simulink model "PV_MODEL4"  (R2023a)
settings: Solver=ode23tb  StartTime=0.0  StopTime=1  RelTol=1e-3
PreLoadFcn:
  | Nss=2;
  | Npp=2;
  | Ki=0.015;
  | Kv=-.1;
  | Tn=25;
  | Vocn=32.9;
  | Iscn=8.21;
  | Rs=.001;
  | Ipvn=8.214;
  | k= (1.38)*(1e-23);
  | Tn=298.15;
  | Gn=1000;
  | a=1.3;
  | q= (1.60) * (1e-19);
  | Ns=54;
  | Rp=600.405;Nss=2;
  | Npp=2;
  | Ki=0.015;
  | Kv=-.1;
  | Tn=25;
  | Vocn=32.9;
  | Iscn=8.21;
  | Rs=.001;
  | Ipvn=8.214;
  | k= (1.38)*(1e-23);
  | Tn=298.15;
  | Gn=1000;
  | a=1.3;
  | q= (1.60) * (1e-19);
  | Ns=54;
  | Rp=600.405;
libraries: spsSeriesRLCBranchLib x4, powerlib_extras x2, spsVoltageMeasurementLib x2, spsCurrentMeasurementLib x1, spsDiodeLib x1, spsIGBTLib x1, simulink x1, spsPVArrayLib x1, sps_lib x1
settings Model: Creator=dell  LastModifiedBy=ankit
settings SolverCC: AlgebraicLoopSolver=TrustRegion
settings DataIOCC: LimitDataPoints=on  SaveFormat=Array  SignalLoggingSaveFormat=ModelDataLogs  ReturnWorkspaceOutputs=off
settings OptimizationCC: BlockReduction=off  BooleanDataType=off  LifeSpan=inf
settings DebuggingCC: SaveWithParameterizedLinksMsg=none  UnderspecifiedInitializationDetection=Classic  MergeDetectMultiDrivingBlocksExec=none  SignalResolutionControl=TryResolveAllWithWarning  MultiTaskDSMMsg=warning  MultiTaskCondExecSysMsg=none  UnconnectedInputMsg=warning  UnconnectedOutputMsg=warning  UnconnectedLineMsg=warning  StateNameClashWarn=warning  SFUnexpectedBacktrackingDiag=warning  SFNoUnconditionalDefaultTransitionDiag=warning  SFExecutionAtInitializationDiag=none  ArithmeticOperatorsInVariantConditions=warning
settings HardwareCC: ProdBitPerPointer=32  ProdBitPerSizeT=32  ProdBitPerPtrDiffT=32  ProdLargestAtomicFloat=None  ProdIntDivRoundTo=Undefined  ProdEndianess=Unspecified  ProdWordSize=32  ProdHWDeviceType=32-bit Generic  TargetUnknown=on
settings ModelReferenceCC: PropagateSignalLabelsOutOfModel=off
settings SFSimCC: SimUseLocalCustomCode=off  CustomCodeUndefinedFunction=UseInterfaceOnly
settings RTWCC: RTWUseLocalCustomCode=off
settings CodeAppCC: StateflowObjectComments=on
settings GRTTargetCC: TargetLangStandard=C89/C90 (ANSI)
settings ConfigComp: CovMetricSettings=dw  CovSaveCumulativeToWorkspaceVar=on  CovSaveSingleToWorkspaceVar=on  CovExternalEMLEnable=off
settings SimscapeCC: SimscapeNormalizeSystem=off

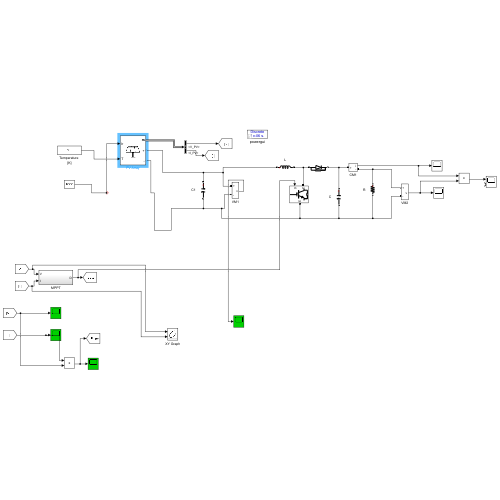
[thumbnail: Simulink's stored preview of the top-level diagram]
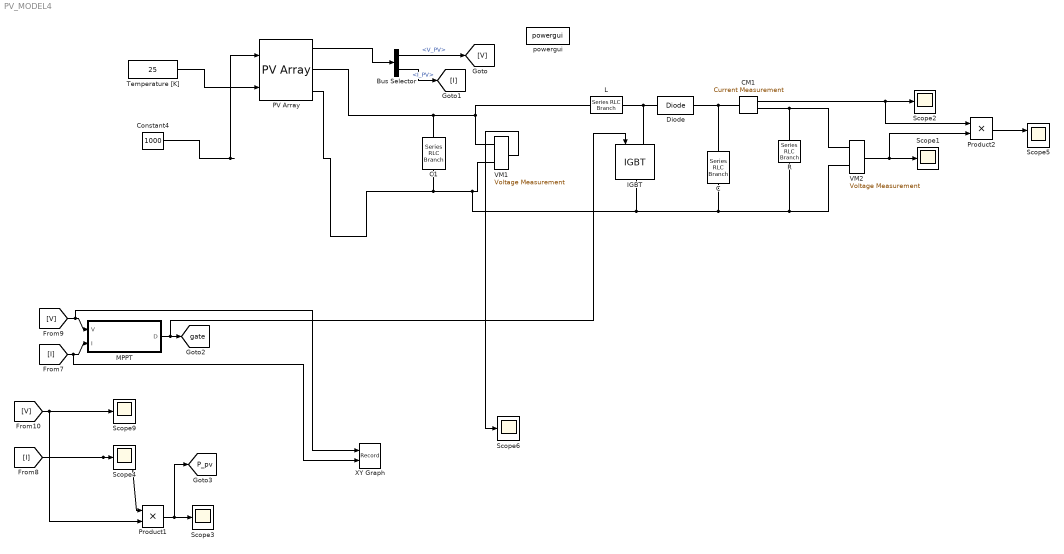
== system PV_MODEL4 ==
  Bus Selector : BusSelector  OutputSignals=V_PV,I_PV
  C : spsSeriesRLCBranchLib/Series RLC Branch  LConnTagsString=__new0  RConnTagsString=__new0  BranchType=C  Resistance=0.01  Inductance=1.0  SetiL0=off  InitialCurrent=0  Capacitance=20e-6  Setx0=off  InitialVoltage=200  Measurements=None
  C1 : spsSeriesRLCBranchLib/Series RLC Branch  LConnTagsString=__new0  RConnTagsString=__new0  BranchType=C  Resistance=0.01  Inductance=1.0  SetiL0=off  InitialCurrent=0  Capacitance=10e-6  Setx0=off  InitialVoltage=200  Measurements=None
  CM1 : spsCurrentMeasurementLib/Current Measurement  Tag=PoWeRsYsTeMmEaSuReMeNt  PhasorSimulation=off  OutputType=Magnitude  PSBequivalent=0
      settings: AttributesFormatString=\n
  Constant4 : Constant  Value=1000
  Diode : spsDiodeLib/Diode  Ron=0.001  Lon=0  Vf=0.8  IC=0  UseSnubber=off  Rs=500  Cs=250e-9  Measurements=off
      settings: AttributesFormatString=\n
  IGBT : spsIGBTLib/IGBT  Ron=0.001  Lon=0  Vf=1  Tf=1e-6  Tt=2e-6  IC=0  Rs=1e5  Cs=inf  Measurements=off
  L : spsSeriesRLCBranchLib/Series RLC Branch  LConnTagsString=__new0  RConnTagsString=__new0  BranchType=L  Resistance=1.0  Inductance=3e-3  SetiL0=off  InitialCurrent=0  Capacitance=1.0  Setx0=off  InitialVoltage=0  Measurements=None
  MPPT : Subsystem
  PV Array : spsPVArrayLib/PV Array  Npar=2  Nser=2  PlotType=array @ 1000 W/m2 & specified temperatures  S_vec="[ 1000  500  100 ]"  Temp_C_vec="[ 25 25  ]"  ModuleName=User-defined  PlotWhenSelected=off  Pm=213.15  Ncell=60  Voc=32.8  Isc=8.21  Vm=29  Im=7.35  beta_Voc_pc=-0.36099  alpha_Isc_pc=0.102  beta_Voc=-0.1184  alpha_Isc=0.0083742  IL=8.2101  I0=1.1241e-09  nI=1.0005  Rsh=67.4422  Rs=0.17921  RobustModel=off  RobustCellTemperature=313.3991  BAL=on  Tc=1e-6  Tfilter=5e-5
  Product1 : Product  RndMeth=Zero
  Product2 : Product  RndMeth=Zero
  R : spsSeriesRLCBranchLib/Series RLC Branch  LConnTagsString=__new0  RConnTagsString=__new0  BranchType=R  Resistance=100  Inductance=1.0  SetiL0=off  InitialCurrent=0  Capacitance=1.0  Setx0=off  InitialVoltage=0  Measurements=None
  Scope{1..4,6,9} (6 alike) : Scope
  Scope5 : Scope  NumInputPorts=2
  Temperature [K] : Constant  Value=25
  VM1 : spsVoltageMeasurementLib/Voltage Measurement  Tag=PoWeRsYsTeMmEaSuReMeNt  PhasorSimulation=off  OutputType=Magnitude  PSBequivalent=0
  VM2 : spsVoltageMeasurementLib/Voltage Measurement  Tag=PoWeRsYsTeMmEaSuReMeNt  PhasorSimulation=off  OutputType=Magnitude  PSBequivalent=0
  XY Graph : Record  FileSettingsInternal="{\"entries\":[{\"content\":{\"excelSettings\":{\"content\":{},\"type\":\"Streamout.ExcelSettings\"}},\"type\":\"Streamout.FileSettingStorage\",\"uuid\":\"703f23f3-b502-4b8b-bb57-5ac5596cb9ef\"}],\"packageUris\":[\"http://schema.mathworks.com/mf0/streamout_blocks/R2020a\"],\"version\":\"1.0\"}"  Layout=[1 1]  SignalsInternal="{\"entries\":[{\"content\":{\"signals\":[{\"content\":{\"blockPath\":[\"PV_MODEL4/XY Graph\"],\"dimensions\":[1],\"domain\":\"PV_MODEL4/XY Graph\",\"lineColor\":\"#77ac30\",\"plots\":[1],\"port\":1,\"sid\":[\"\"],\"signalID\":3832,\"signalName\":\"From9\"},\"type\":\"RecordBlkView.Signal\",\"uuid\":\"d7ffbdd2-4cad-46f6-af63-4d1a62489c55\"},{\"content\":{\"blockPath\":[\"PV_MODEL4/XY Graph\"],\"dimensions\":[1],\"domain\":\"PV_MODEL4/XY Graph\",\"lineColor\":\"#4dbeee\",\"plots\":[1],\"port\":2,\"sid\":[\"\"],\"signalID\":3836,\"signalName\":\"From7\"},\"type\":\"RecordBlkView.Signal\",\"uuid\":\"233419f2-317b-4a01-aaa1-3c486f545b7b\"}]},\"type\":\"RecordBlkView.InputSignals\",\"uuid\":\"455b5cee-85e1-48e0-afff-2121fab88297\"}],\"packageUris\":[\"http://schema.mathworks.com/mf0/streamout_blocks/R2020a\"],\"version\":\"1.0\"}"  VisualizationBindings="{\"xyplotplugin\":{\"info\":[{\"series\":[{\"bindingParametersList\":[{\"parameter\":\"X-Axis\",\"signalID\":3832,\"signalName\":\"From9\"},{\"parameter\":\"Y-Axis\",\"signalID\":3836,\"signalName\":\"From7\"}],\"seriesID\":2784}],\"subplotID\":1}]}}"  CompatibilityTag=XY  st=-1
  powergui : sps_lib/powergui  SimulationMode=Discrete  SampleTime=1e-6  frequency=60  Iterations=50  frequencyindice=0  Pbase=100e6  ErrMax=1e-4  UnitsV=kV  UnitsW=MW  buscounter=0  FunctionMessages=off  echomessages=off  EnableUseOfTLC=off  CurrentSourceSwitches=off  DisableSnubberDevices=off  DisableRonSwitches=off  DisableVfSwitches=off  DisplayEquations=off  AutomaticDiscreteSolvers=off  SolverType=Tustin  Interpol=off  ExternalGateDelay=off  methode=off  Ts=0  x0status=blocks  SPID=off  SwTol=0  HookPort=off  NonlinearTolerance=1e-4  nMaxIteration=100  ContinueOnMaxIteration=off  RestoreLinks=warning  ResistiveCurrentMeasurement=off  Frange=[0:2:500]  Ylog=off  Xlog=on  ShowGrid=off  save=off  variable=ZData  structure=0  ZoomFFT=on  StartTime=0.0  cycles=1  DisplayStyle=1  fundamental=60  FreqAxis=off  MaxFrequency=1000  frequencyindicesteady=1  RmsSteady=1  display=off
  tag scope: P_pv=global, gate=global
  wires:
  Temperature [K]/1 -> PV Array/2
  [I] -> XY Graph/2, MPPT/2(I)
  [V] -> XY Graph/1, MPPT/1(V)
  Product1/1 -> [P_pv], Scope3/1
  [I] -> Product1/1, Scope4/1
  [V] -> Product1/2, Scope9/1
  CM1/1 -> Scope2/1, Product2/1
  VM2/1 -> Scope1/1, Product2/2
  MPPT/1(D) -> IGBT/1, [gate]
  Product2/1 -> Scope5/1
  VM1/1 -> Scope6/1
  Constant4/1 -> PV Array/1
  PV Array/1 -> Bus Selector/1
  Bus Selector/1 -> [V]  "<V_PV>"
  Bus Selector/2 -> [I]  "<I_PV>"
  connections:
  C1/LConn1 -- PV Array/RConn1 -- VM1/LConn1 -- L/LConn1
  IGBT/RConn1 -- PV Array/RConn2 -- C1/RConn1 -- VM1/LConn2 -- C/RConn1 -- VM2/LConn2 -- R/RConn1
  C/LConn1 -- Diode/RConn1 -- CM1/LConn1
  Diode/LConn1 -- IGBT/LConn1 -- L/RConn1
  CM1/RConn1 -- R/LConn1 -- VM2/LConn1

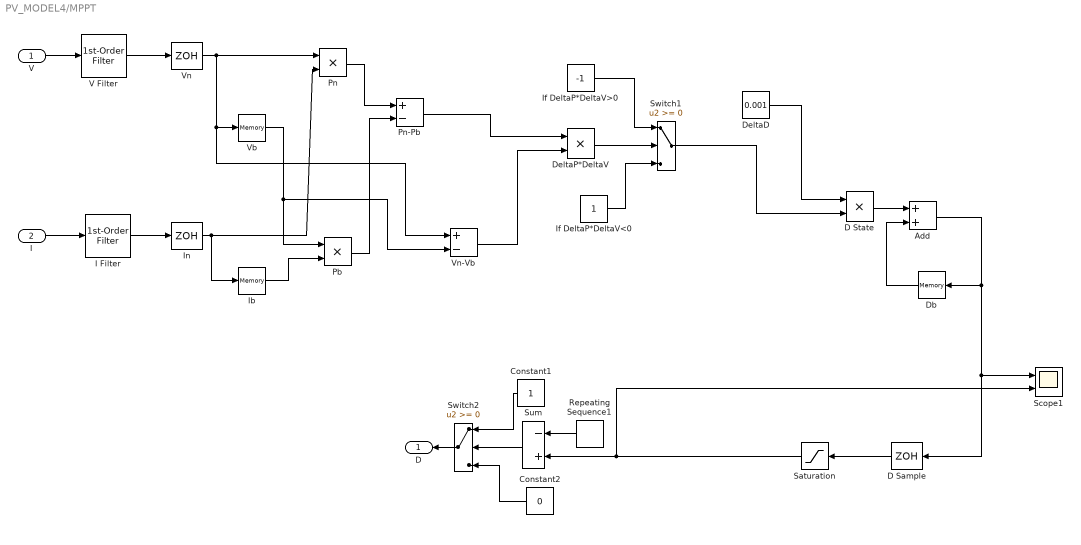
== system PV_MODEL4/MPPT ==
  V : Inport
  I : Inport  Port=2
  Add : Sum
  Constant1 : Constant  SampleTime=-1
  Constant2 : Constant  Value=0  SampleTime=-1
  D Sample : ZeroOrderHold  SampleTime=1e-4
  D State : Product  RndMeth=Zero
  Db : Memory  InheritSampleTime=on  LinearizeAsDelay=on
  DeltaD : Constant  Value=0.001
  DeltaP*DeltaV : Product  RndMeth=Zero
  I Filter : powerlib_extras/Control  Blocks/1st-Order  Filter  FilterType=Lowpass  Tc=1e-3  Initialize=off  Vac_Init=[0.8 -25 60]  Vdc_Init=-0.4  PlotResponse=off  param1=[1 500 1]
  Ib : Memory  InheritSampleTime=on  LinearizeAsDelay=on
  If DeltaP*DeltaV<0 : Constant
  If DeltaP*DeltaV>0 : Constant  Value=-1
  In : ZeroOrderHold  SampleTime=1e-4
  Pb : Product  RndMeth=Zero
  Pn : Product  RndMeth=Zero
  Pn-Pb : Sum  Inputs=+-
  Repeating Sequence1 : simulink/Sources/Repeating Sequence  rep_seq_t=[0 50e-6]  rep_seq_y=[0 1]
  Saturation : Saturate  UpperLimit=0.8  LowerLimit=0
  Scope1 : Scope  NumInputPorts=2
  Sum : Sum  Inputs=-+  SaturateOnIntegerOverflow=on
  Switch1 : Switch  SaturateOnIntegerOverflow=off  InputSameDT=off
  Switch2 : Switch  SaturateOnIntegerOverflow=off  InputSameDT=off
  V Filter : powerlib_extras/Control  Blocks/1st-Order  Filter  FilterType=Lowpass  Tc=1e-3  Initialize=off  Vac_Init=[0.8 -25 60]  Vdc_Init=-0.4  PlotResponse=off  param1=[1 500 1]
  Vb : Memory  InheritSampleTime=on  LinearizeAsDelay=on
  Vn : ZeroOrderHold  SampleTime=1e-4
  Vn-Vb : Sum  Inputs=+-
  D : Outport
  wires:
  V/1 -> V Filter/1
  I/1 -> I Filter/1
  V Filter/1 -> Vn/1
  I Filter/1 -> In/1
  In/1 -> Ib/1, Pn/2
  Vn/1 -> Pn/1, Vb/1, Vn-Vb/1
  Ib/1 -> Pb/2
  Vb/1 -> Pb/1, Vn-Vb/2
  Pn/1 -> Pn-Pb/1
  Pb/1 -> Pn-Pb/2
  D State/1 -> Add/1
  Constant2/1 -> Switch2/3
  Constant1/1 -> Switch2/1
  Sum/1 -> Switch2/2
  Repeating Sequence1/1 -> Sum/1
  Add/1 -> Db/1, D Sample/1, Scope1/1
  Switch2/1 -> D/1
  Db/1 -> Add/2
  D Sample/1 -> Saturation/1
  Pn-Pb/1 -> DeltaP*DeltaV/1
  Vn-Vb/1 -> DeltaP*DeltaV/2
  DeltaP*DeltaV/1 -> Switch1/2
  If DeltaP*DeltaV>0/1 -> Switch1/1
  If DeltaP*DeltaV<0/1 -> Switch1/3
  Switch1/1 -> D State/2
  DeltaD/1 -> D State/1
  Saturation/1 -> Sum/2, Scope1/2
